simulink model "montaje"  (R2022b)
settings: Solver=VariableStepAuto  StartTime=0.0  StopTime=10.0  RelTol=1e-3
values from neighbouring files (symbols this model uses):
  B = 0.2    [conf.m]
  g = 9.8    [conf.m]
  J = 0.006    [conf.m]
  L = 0.5    [conf.m]
  M = 1    [conf.m]
  Ref = pi/4    (= 0.785398163397)    [conf.m]
undefined symbols (not defined in the file or in its folder): difuso10
libraries: fuzblock x1
settings Model: Creator=Admin  LastModifiedBy=David
settings OptimizationCC: ReuseModelBlockBuffer=on

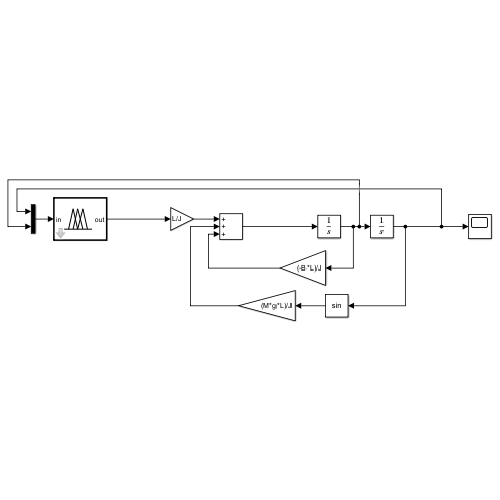
[thumbnail: Simulink's stored preview of the top-level diagram]
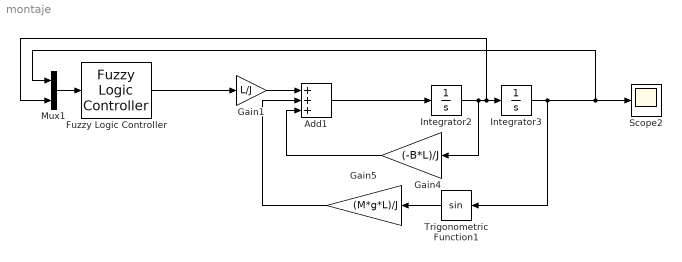
== system montaje ==
  Add1 : Sum  Inputs=+++
  Fuzzy Logic Controller : fuzblock/Fuzzy Logic  Controller  FIS=[difuso10]  OutputSampleNumber=101  DataType=double  FuzzifiedInputs=off  RuleFiringStrengths=off  RuleOutputs=off  AggregatedOutputs=off  SimulateUsing=Interpreted execution  OutOfRangeInputValueMessage=warning  NoRuleFiredMessage=warning  EmptyOutputFuzzySetMessage=warning
  Gain1 : Gain  Gain=L/J
  Gain4 : Gain  Gain=(-B*L)/J
  Gain5 : Gain  Gain=(M*g*L)/J
  Integrator2 : Integrator
  Integrator3 : Integrator  InitialCondition=Ref
  Mux1 : Mux  Inputs=2
  Scope2 : Scope
  Trigonometric Function1 : Trigonometry
  wires:
  Gain5/1 -> Add1/2
  Integrator2/1 -> Gain4/1, Mux1/2, Integrator3/1
  Integrator3/1 -> Mux1/1, Scope2/1, Trigonometric Function1/1
  Trigonometric Function1/1 -> Gain5/1
  Add1/1 -> Integrator2/1
  Gain4/1 -> Add1/3
  Gain1/1 -> Add1/1
  Fuzzy Logic Controller/1 -> Gain1/1
  Mux1/1 -> Fuzzy Logic Controller/1
